simulink model "ProgramaPiero"  (R2024b)
settings: Solver=VariableStepAuto  StartTime=0.0  StopTime=10.0  RelTol=1e-3
settings Model: Creator=Laura  LastModifiedBy=Laura

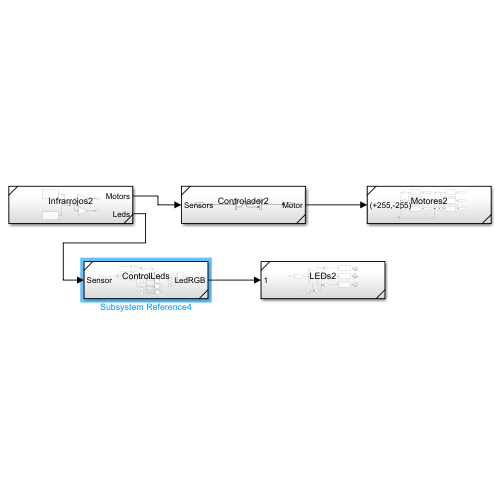
[thumbnail: Simulink's stored preview of the top-level diagram]
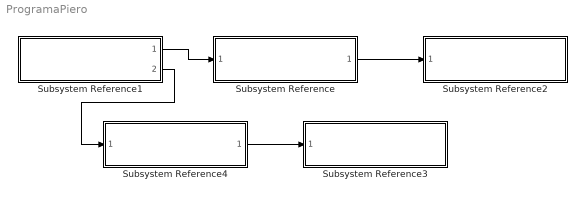
== system ProgramaPiero ==
  Subsystem Reference : Subsystem  ReferencedSubsystem=Controlador2
  Subsystem Reference1 : Subsystem  ReferencedSubsystem=Infrarrojos2
  Subsystem Reference2 : Subsystem  ReferencedSubsystem=Motores2
  Subsystem Reference3 : Subsystem  ReferencedSubsystem=LEDs2
  Subsystem Reference4 : Subsystem  ReferencedSubsystem=ControlLeds
  wires:
  Subsystem Reference1/1 -> Subsystem Reference/1
  Subsystem Reference/1 -> Subsystem Reference2/1
  Subsystem Reference4/1 -> Subsystem Reference3/1
  Subsystem Reference1/2 -> Subsystem Reference4/1
